simulink model "Sine_Wave_question2"  (R2023b)
settings: Solver=FixedStepAuto  StartTime=0.0  StopTime=0.04  RelTol=1e-3
settings Model: Creator=Pranav  LastModifiedBy=Pranav

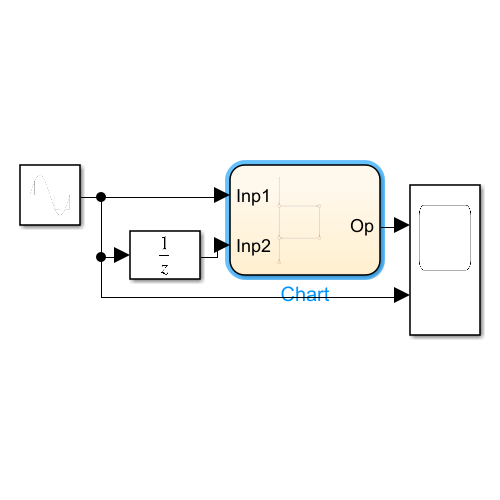
[thumbnail: Simulink's stored preview of the top-level diagram]
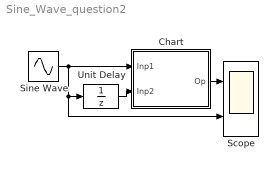
== system Sine_Wave_question2 ==
  Chart : Stateflow chart  TreatAsAtomicUnit=on
  Scope : Scope  NumInputPorts=2
  Sine Wave : Sin  Frequency=314  SampleTime=5e-5
  Unit Delay : UnitDelay  SampleTime=-1  HasFrameUpgradeWarning=on
  wires:
  Unit Delay/1 -> Chart/2(Inp2)
  Chart/1(Op) -> Scope/1
  Sine Wave/1 -> Scope/2, Unit Delay/1, Chart/1(Inp1)

== stateflow chart Sine_Wave_question2/Chart ==
  (default) -> (junction 1)
  (junction 1) -> (junction 3) [order 1] : [Inp1>Inp2]
  (junction 1) -> (junction 12) [order 2] : {Op=-1;}
  (junction 3) -> (junction 8) : {Op=1;}
  (junction 8) -> (junction 12)
  (junction 12) -> (junction 15)
  data: Inp1 input; Inp2 input; Op output
